simulink model "test"  (R2015a)
settings: Solver=ode45  StartTime=0.0  StopTime=380000  RelTol=1e-3
InitFcn:
  | %% DSPBuilder Start
  | alt_dspbuilder_update_model(bdroot)
  | %% DSPBuilder End
libraries: allblocks_alteradspbuilder2 x2155
(part 4 of 24)

== system test/octave2/compare_descriptor/get_distance5 ==
  hist_in1 : Inport
  hist_in2 : Inport  Port=2
  clken : Inport  Port=3
  BusSplitter : Subsystem
  BusSplitter1 : Subsystem
  Parallel Adder Subtractor : allblocks_alteradspbuilder2/Parallel Adder Subtractor  number_of_inputs=8  direction=+  use_pipeline=on  pipeline_display=3  phase_selection=1  use_ena=on  use_aclr=off  allowFloatingPointOverride=on  logOutputs=off  logFile=C:\Users\ASUS\Desktop\sift_fpga_final\Octave_2\tb_test\test_octave2_compare%5Fdescriptor_get%5Fdistance5_Parallel+Adder+Subtractor.fixedpointlog
  sub_GradOrian : Subsystem
  sub_GradOrian1 : Subsystem
  sub_GradOrian2 : Subsystem
  sub_GradOrian3 : Subsystem
  sub_GradOrian4 : Subsystem
  sub_GradOrian5 : Subsystem
  sub_GradOrian6 : Subsystem
  sub_GradOrian7 : Subsystem
  distance_out : Outport
  wires:
  hist_in2/1 -> [hist_in2]
  hist_in1/1 -> [hist_in1]
  [hist_in1] -> BusSplitter/1(data_in)
  [hist_in2] -> BusSplitter1/1(data_in)
  BusSplitter/1(bin1) -> [bin_11]
  BusSplitter/2(bin2) -> [bin_12]
  BusSplitter/3(bin3) -> [bin_13]
  BusSplitter/4(bin4) -> [bin_14]
  BusSplitter/5(bin5) -> [bin_15]
  BusSplitter/6(bin6) -> [bin_16]
  BusSplitter/7(bin7) -> [bin_17]
  BusSplitter/8(bin8) -> [bin_18]
  BusSplitter1/1(bin1) -> [bin_21]
  BusSplitter1/2(bin2) -> [bin_22]
  BusSplitter1/3(bin3) -> [bin_23]
  BusSplitter1/4(bin4) -> [bin_24]
  BusSplitter1/5(bin5) -> [bin_25]
  BusSplitter1/6(bin6) -> [bin_26]
  BusSplitter1/7(bin7) -> [bin_27]
  BusSplitter1/8(bin8) -> [bin_28]
  [bin_21] -> sub_GradOrian/2(bin2)
  [bin_11] -> sub_GradOrian/1(bin1)
  clken/1 -> [clken]
  [clken] -> sub_GradOrian/3(clken)
  sub_GradOrian/1(sub_bin) -> [sub_bin1]
  [bin_22] -> sub_GradOrian1/2(bin2)
  [bin_12] -> sub_GradOrian1/1(bin1)
  [clken] -> sub_GradOrian1/3(clken)
  sub_GradOrian1/1(sub_bin) -> [sub_bin2]
  [bin_23] -> sub_GradOrian2/2(bin2)
  [bin_13] -> sub_GradOrian2/1(bin1)
  [clken] -> sub_GradOrian2/3(clken)
  sub_GradOrian2/1(sub_bin) -> [sub_bin3]
  [bin_24] -> sub_GradOrian3/2(bin2)
  [bin_14] -> sub_GradOrian3/1(bin1)
  [clken] -> sub_GradOrian3/3(clken)
  sub_GradOrian3/1(sub_bin) -> [sub_bin4]
  [bin_25] -> sub_GradOrian4/2(bin2)
  [bin_15] -> sub_GradOrian4/1(bin1)
  [clken] -> sub_GradOrian4/3(clken)
  sub_GradOrian4/1(sub_bin) -> [sub_bin5]
  [bin_26] -> sub_GradOrian5/2(bin2)
  [bin_16] -> sub_GradOrian5/1(bin1)
  [clken] -> sub_GradOrian5/3(clken)
  sub_GradOrian5/1(sub_bin) -> [sub_bin6]
  [bin_27] -> sub_GradOrian6/2(bin2)
  [bin_17] -> sub_GradOrian6/1(bin1)
  [clken] -> sub_GradOrian6/3(clken)
  sub_GradOrian6/1(sub_bin) -> [sub_bin7]
  [bin_28] -> sub_GradOrian7/2(bin2)
  [bin_18] -> sub_GradOrian7/1(bin1)
  [clken] -> sub_GradOrian7/3(clken)
  sub_GradOrian7/1(sub_bin) -> [sub_bin8]
  [sub_bin1] -> Parallel Adder Subtractor/1
  [sub_bin2] -> Parallel Adder Subtractor/2
  [sub_bin3] -> Parallel Adder Subtractor/3
  [sub_bin4] -> Parallel Adder Subtractor/4
  [sub_bin5] -> Parallel Adder Subtractor/5
  [sub_bin6] -> Parallel Adder Subtractor/6
  [sub_bin7] -> Parallel Adder Subtractor/7
  [sub_bin8] -> Parallel Adder Subtractor/8
  [clken] -> Parallel Adder Subtractor/9
  Parallel Adder Subtractor/1 -> [distance_out]
  [distance_out] -> distance_out/1

== system test/octave2/compare_descriptor/get_distance6 ==
  hist_in1 : Inport
  hist_in2 : Inport  Port=2
  clken : Inport  Port=3
  BusSplitter : Subsystem
  BusSplitter1 : Subsystem
  Parallel Adder Subtractor : allblocks_alteradspbuilder2/Parallel Adder Subtractor  number_of_inputs=8  direction=+  use_pipeline=on  pipeline_display=3  phase_selection=1  use_ena=on  use_aclr=off  allowFloatingPointOverride=on  logOutputs=off  logFile=C:\Users\ASUS\Desktop\sift_fpga_final\Octave_2\tb_test\test_octave2_compare%5Fdescriptor_get%5Fdistance6_Parallel+Adder+Subtractor.fixedpointlog
  sub_GradOrian : Subsystem
  sub_GradOrian1 : Subsystem
  sub_GradOrian2 : Subsystem
  sub_GradOrian3 : Subsystem
  sub_GradOrian4 : Subsystem
  sub_GradOrian5 : Subsystem
  sub_GradOrian6 : Subsystem
  sub_GradOrian7 : Subsystem
  distance_out : Outport
  wires:
  hist_in2/1 -> [hist_in2]
  hist_in1/1 -> [hist_in1]
  [hist_in1] -> BusSplitter/1(data_in)
  [hist_in2] -> BusSplitter1/1(data_in)
  BusSplitter/1(bin1) -> [bin_11]
  BusSplitter/2(bin2) -> [bin_12]
  BusSplitter/3(bin3) -> [bin_13]
  BusSplitter/4(bin4) -> [bin_14]
  BusSplitter/5(bin5) -> [bin_15]
  BusSplitter/6(bin6) -> [bin_16]
  BusSplitter/7(bin7) -> [bin_17]
  BusSplitter/8(bin8) -> [bin_18]
  BusSplitter1/1(bin1) -> [bin_21]
  BusSplitter1/2(bin2) -> [bin_22]
  BusSplitter1/3(bin3) -> [bin_23]
  BusSplitter1/4(bin4) -> [bin_24]
  BusSplitter1/5(bin5) -> [bin_25]
  BusSplitter1/6(bin6) -> [bin_26]
  BusSplitter1/7(bin7) -> [bin_27]
  BusSplitter1/8(bin8) -> [bin_28]
  [bin_21] -> sub_GradOrian/2(bin2)
  [bin_11] -> sub_GradOrian/1(bin1)
  clken/1 -> [clken]
  [clken] -> sub_GradOrian/3(clken)
  sub_GradOrian/1(sub_bin) -> [sub_bin1]
  [bin_22] -> sub_GradOrian1/2(bin2)
  [bin_12] -> sub_GradOrian1/1(bin1)
  [clken] -> sub_GradOrian1/3(clken)
  sub_GradOrian1/1(sub_bin) -> [sub_bin2]
  [bin_23] -> sub_GradOrian2/2(bin2)
  [bin_13] -> sub_GradOrian2/1(bin1)
  [clken] -> sub_GradOrian2/3(clken)
  sub_GradOrian2/1(sub_bin) -> [sub_bin3]
  [bin_24] -> sub_GradOrian3/2(bin2)
  [bin_14] -> sub_GradOrian3/1(bin1)
  [clken] -> sub_GradOrian3/3(clken)
  sub_GradOrian3/1(sub_bin) -> [sub_bin4]
  [bin_25] -> sub_GradOrian4/2(bin2)
  [bin_15] -> sub_GradOrian4/1(bin1)
  [clken] -> sub_GradOrian4/3(clken)
  sub_GradOrian4/1(sub_bin) -> [sub_bin5]
  [bin_26] -> sub_GradOrian5/2(bin2)
  [bin_16] -> sub_GradOrian5/1(bin1)
  [clken] -> sub_GradOrian5/3(clken)
  sub_GradOrian5/1(sub_bin) -> [sub_bin6]
  [bin_27] -> sub_GradOrian6/2(bin2)
  [bin_17] -> sub_GradOrian6/1(bin1)
  [clken] -> sub_GradOrian6/3(clken)
  sub_GradOrian6/1(sub_bin) -> [sub_bin7]
  [bin_28] -> sub_GradOrian7/2(bin2)
  [bin_18] -> sub_GradOrian7/1(bin1)
  [clken] -> sub_GradOrian7/3(clken)
  sub_GradOrian7/1(sub_bin) -> [sub_bin8]
  [sub_bin1] -> Parallel Adder Subtractor/1
  [sub_bin2] -> Parallel Adder Subtractor/2
  [sub_bin3] -> Parallel Adder Subtractor/3
  [sub_bin4] -> Parallel Adder Subtractor/4
  [sub_bin5] -> Parallel Adder Subtractor/5
  [sub_bin6] -> Parallel Adder Subtractor/6
  [sub_bin7] -> Parallel Adder Subtractor/7
  [sub_bin8] -> Parallel Adder Subtractor/8
  [clken] -> Parallel Adder Subtractor/9
  Parallel Adder Subtractor/1 -> [distance_out]
  [distance_out] -> distance_out/1

== system test/octave2/compare_descriptor/get_distance7 ==
  hist_in1 : Inport
  hist_in2 : Inport  Port=2
  clken : Inport  Port=3
  BusSplitter : Subsystem
  BusSplitter1 : Subsystem
  Parallel Adder Subtractor : allblocks_alteradspbuilder2/Parallel Adder Subtractor  number_of_inputs=8  direction=+  use_pipeline=on  pipeline_display=3  phase_selection=1  use_ena=on  use_aclr=off  allowFloatingPointOverride=on  logOutputs=off  logFile=C:\Users\ASUS\Desktop\sift_fpga_final\Octave_2\tb_test\test_octave2_compare%5Fdescriptor_get%5Fdistance7_Parallel+Adder+Subtractor.fixedpointlog
  sub_GradOrian : Subsystem
  sub_GradOrian1 : Subsystem
  sub_GradOrian2 : Subsystem
  sub_GradOrian3 : Subsystem
  sub_GradOrian4 : Subsystem
  sub_GradOrian5 : Subsystem
  sub_GradOrian6 : Subsystem
  sub_GradOrian7 : Subsystem
  distance_out : Outport
  wires:
  hist_in2/1 -> [hist_in2]
  hist_in1/1 -> [hist_in1]
  [hist_in1] -> BusSplitter/1(data_in)
  [hist_in2] -> BusSplitter1/1(data_in)
  BusSplitter/1(bin1) -> [bin_11]
  BusSplitter/2(bin2) -> [bin_12]
  BusSplitter/3(bin3) -> [bin_13]
  BusSplitter/4(bin4) -> [bin_14]
  BusSplitter/5(bin5) -> [bin_15]
  BusSplitter/6(bin6) -> [bin_16]
  BusSplitter/7(bin7) -> [bin_17]
  BusSplitter/8(bin8) -> [bin_18]
  BusSplitter1/1(bin1) -> [bin_21]
  BusSplitter1/2(bin2) -> [bin_22]
  BusSplitter1/3(bin3) -> [bin_23]
  BusSplitter1/4(bin4) -> [bin_24]
  BusSplitter1/5(bin5) -> [bin_25]
  BusSplitter1/6(bin6) -> [bin_26]
  BusSplitter1/7(bin7) -> [bin_27]
  BusSplitter1/8(bin8) -> [bin_28]
  [bin_21] -> sub_GradOrian/2(bin2)
  [bin_11] -> sub_GradOrian/1(bin1)
  clken/1 -> [clken]
  [clken] -> sub_GradOrian/3(clken)
  sub_GradOrian/1(sub_bin) -> [sub_bin1]
  [bin_22] -> sub_GradOrian1/2(bin2)
  [bin_12] -> sub_GradOrian1/1(bin1)
  [clken] -> sub_GradOrian1/3(clken)
  sub_GradOrian1/1(sub_bin) -> [sub_bin2]
  [bin_23] -> sub_GradOrian2/2(bin2)
  [bin_13] -> sub_GradOrian2/1(bin1)
  [clken] -> sub_GradOrian2/3(clken)
  sub_GradOrian2/1(sub_bin) -> [sub_bin3]
  [bin_24] -> sub_GradOrian3/2(bin2)
  [bin_14] -> sub_GradOrian3/1(bin1)
  [clken] -> sub_GradOrian3/3(clken)
  sub_GradOrian3/1(sub_bin) -> [sub_bin4]
  [bin_25] -> sub_GradOrian4/2(bin2)
  [bin_15] -> sub_GradOrian4/1(bin1)
  [clken] -> sub_GradOrian4/3(clken)
  sub_GradOrian4/1(sub_bin) -> [sub_bin5]
  [bin_26] -> sub_GradOrian5/2(bin2)
  [bin_16] -> sub_GradOrian5/1(bin1)
  [clken] -> sub_GradOrian5/3(clken)
  sub_GradOrian5/1(sub_bin) -> [sub_bin6]
  [bin_27] -> sub_GradOrian6/2(bin2)
  [bin_17] -> sub_GradOrian6/1(bin1)
  [clken] -> sub_GradOrian6/3(clken)
  sub_GradOrian6/1(sub_bin) -> [sub_bin7]
  [bin_28] -> sub_GradOrian7/2(bin2)
  [bin_18] -> sub_GradOrian7/1(bin1)
  [clken] -> sub_GradOrian7/3(clken)
  sub_GradOrian7/1(sub_bin) -> [sub_bin8]
  [sub_bin1] -> Parallel Adder Subtractor/1
  [sub_bin2] -> Parallel Adder Subtractor/2
  [sub_bin3] -> Parallel Adder Subtractor/3
  [sub_bin4] -> Parallel Adder Subtractor/4
  [sub_bin5] -> Parallel Adder Subtractor/5
  [sub_bin6] -> Parallel Adder Subtractor/6
  [sub_bin7] -> Parallel Adder Subtractor/7
  [sub_bin8] -> Parallel Adder Subtractor/8
  [clken] -> Parallel Adder Subtractor/9
  Parallel Adder Subtractor/1 -> [distance_out]
  [distance_out] -> distance_out/1

== system test/octave2/compare_descriptor/get_distance8 ==
  hist_in1 : Inport
  hist_in2 : Inport  Port=2
  clken : Inport  Port=3
  BusSplitter : Subsystem
  BusSplitter1 : Subsystem
  Parallel Adder Subtractor : allblocks_alteradspbuilder2/Parallel Adder Subtractor  number_of_inputs=8  direction=+  use_pipeline=on  pipeline_display=3  phase_selection=1  use_ena=on  use_aclr=off  allowFloatingPointOverride=on  logOutputs=off  logFile=C:\Users\ASUS\Desktop\sift_fpga_final\Octave_2\tb_test\test_octave2_compare%5Fdescriptor_get%5Fdistance8_Parallel+Adder+Subtractor.fixedpointlog
  sub_GradOrian : Subsystem
  sub_GradOrian1 : Subsystem
  sub_GradOrian2 : Subsystem
  sub_GradOrian3 : Subsystem
  sub_GradOrian4 : Subsystem
  sub_GradOrian5 : Subsystem
  sub_GradOrian6 : Subsystem
  sub_GradOrian7 : Subsystem
  distance_out : Outport
  wires:
  hist_in2/1 -> [hist_in2]
  hist_in1/1 -> [hist_in1]
  [hist_in1] -> BusSplitter/1(data_in)
  [hist_in2] -> BusSplitter1/1(data_in)
  BusSplitter/1(bin1) -> [bin_11]
  BusSplitter/2(bin2) -> [bin_12]
  BusSplitter/3(bin3) -> [bin_13]
  BusSplitter/4(bin4) -> [bin_14]
  BusSplitter/5(bin5) -> [bin_15]
  BusSplitter/6(bin6) -> [bin_16]
  BusSplitter/7(bin7) -> [bin_17]
  BusSplitter/8(bin8) -> [bin_18]
  BusSplitter1/1(bin1) -> [bin_21]
  BusSplitter1/2(bin2) -> [bin_22]
  BusSplitter1/3(bin3) -> [bin_23]
  BusSplitter1/4(bin4) -> [bin_24]
  BusSplitter1/5(bin5) -> [bin_25]
  BusSplitter1/6(bin6) -> [bin_26]
  BusSplitter1/7(bin7) -> [bin_27]
  BusSplitter1/8(bin8) -> [bin_28]
  [bin_21] -> sub_GradOrian/2(bin2)
  [bin_11] -> sub_GradOrian/1(bin1)
  clken/1 -> [clken]
  [clken] -> sub_GradOrian/3(clken)
  sub_GradOrian/1(sub_bin) -> [sub_bin1]
  [bin_22] -> sub_GradOrian1/2(bin2)
  [bin_12] -> sub_GradOrian1/1(bin1)
  [clken] -> sub_GradOrian1/3(clken)
  sub_GradOrian1/1(sub_bin) -> [sub_bin2]
  [bin_23] -> sub_GradOrian2/2(bin2)
  [bin_13] -> sub_GradOrian2/1(bin1)
  [clken] -> sub_GradOrian2/3(clken)
  sub_GradOrian2/1(sub_bin) -> [sub_bin3]
  [bin_24] -> sub_GradOrian3/2(bin2)
  [bin_14] -> sub_GradOrian3/1(bin1)
  [clken] -> sub_GradOrian3/3(clken)
  sub_GradOrian3/1(sub_bin) -> [sub_bin4]
  [bin_25] -> sub_GradOrian4/2(bin2)
  [bin_15] -> sub_GradOrian4/1(bin1)
  [clken] -> sub_GradOrian4/3(clken)
  sub_GradOrian4/1(sub_bin) -> [sub_bin5]
  [bin_26] -> sub_GradOrian5/2(bin2)
  [bin_16] -> sub_GradOrian5/1(bin1)
  [clken] -> sub_GradOrian5/3(clken)
  sub_GradOrian5/1(sub_bin) -> [sub_bin6]
  [bin_27] -> sub_GradOrian6/2(bin2)
  [bin_17] -> sub_GradOrian6/1(bin1)
  [clken] -> sub_GradOrian6/3(clken)
  sub_GradOrian6/1(sub_bin) -> [sub_bin7]
  [bin_28] -> sub_GradOrian7/2(bin2)
  [bin_18] -> sub_GradOrian7/1(bin1)
  [clken] -> sub_GradOrian7/3(clken)
  sub_GradOrian7/1(sub_bin) -> [sub_bin8]
  [sub_bin1] -> Parallel Adder Subtractor/1
  [sub_bin2] -> Parallel Adder Subtractor/2
  [sub_bin3] -> Parallel Adder Subtractor/3
  [sub_bin4] -> Parallel Adder Subtractor/4
  [sub_bin5] -> Parallel Adder Subtractor/5
  [sub_bin6] -> Parallel Adder Subtractor/6
  [sub_bin7] -> Parallel Adder Subtractor/7
  [sub_bin8] -> Parallel Adder Subtractor/8
  [clken] -> Parallel Adder Subtractor/9
  Parallel Adder Subtractor/1 -> [distance_out]
  [distance_out] -> distance_out/1

== system test/octave2/descriptor/BusSplitter ==
  data_in : Inport
  AltBus : allblocks_alteradspbuilder2/AltBus  BusType=Unsigned Integer  bwl=112  bwr=0  saturate=off  floatingPointInput=on  floatingPointOutput=on  logOutputs=off  logFile=C:\Users\ASUS\Desktop\sift_fpga_final\Octave_2\tb_test\test_octave2_descriptor_BusSplitter_AltBus.fixedpointlog
  AltBus1 : allblocks_alteradspbuilder2/AltBus  BusType=Unsigned Integer  bwl=96  bwr=0  saturate=off  floatingPointInput=on  floatingPointOutput=on  logOutputs=off  logFile=C:\Users\ASUS\Desktop\sift_fpga_final\Octave_2\tb_test\test_octave2_descriptor_BusSplitter_AltBus1.fixedpointlog
  AltBus10 : allblocks_alteradspbuilder2/AltBus  BusType=Unsigned Integer  bwl=16  bwr=0  saturate=off  floatingPointInput=on  floatingPointOutput=on  logOutputs=off  logFile=C:\Users\ASUS\Desktop\sift_fpga_final\Octave_2\tb_test\test_octave2_descriptor_BusSplitter_AltBus10.fixedpointlog
  AltBus11 : allblocks_alteradspbuilder2/AltBus  BusType=Unsigned Integer  bwl=16  bwr=0  saturate=off  floatingPointInput=on  floatingPointOutput=on  logOutputs=off  logFile=C:\Users\ASUS\Desktop\sift_fpga_final\Octave_2\tb_test\test_octave2_descriptor_BusSplitter_AltBus11.fixedpointlog
  AltBus12 : allblocks_alteradspbuilder2/AltBus  BusType=Unsigned Integer  bwl=16  bwr=0  saturate=off  floatingPointInput=on  floatingPointOutput=on  logOutputs=off  logFile=C:\Users\ASUS\Desktop\sift_fpga_final\Octave_2\tb_test\test_octave2_descriptor_BusSplitter_AltBus12.fixedpointlog
  AltBus13 : allblocks_alteradspbuilder2/AltBus  BusType=Unsigned Integer  bwl=16  bwr=0  saturate=off  floatingPointInput=on  floatingPointOutput=on  logOutputs=off  logFile=C:\Users\ASUS\Desktop\sift_fpga_final\Octave_2\tb_test\test_octave2_descriptor_BusSplitter_AltBus13.fixedpointlog
  AltBus2 : allblocks_alteradspbuilder2/AltBus  BusType=Unsigned Integer  bwl=80  bwr=0  saturate=off  floatingPointInput=on  floatingPointOutput=on  logOutputs=off  logFile=C:\Users\ASUS\Desktop\sift_fpga_final\Octave_2\tb_test\test_octave2_descriptor_BusSplitter_AltBus2.fixedpointlog
  AltBus3 : allblocks_alteradspbuilder2/AltBus  BusType=Unsigned Integer  bwl=64  bwr=0  saturate=off  floatingPointInput=on  floatingPointOutput=on  logOutputs=off  logFile=C:\Users\ASUS\Desktop\sift_fpga_final\Octave_2\tb_test\test_octave2_descriptor_BusSplitter_AltBus3.fixedpointlog
  AltBus4 : allblocks_alteradspbuilder2/AltBus  BusType=Unsigned Integer  bwl=48  bwr=0  saturate=off  floatingPointInput=on  floatingPointOutput=on  logOutputs=off  logFile=C:\Users\ASUS\Desktop\sift_fpga_final\Octave_2\tb_test\test_octave2_descriptor_BusSplitter_AltBus4.fixedpointlog
  AltBus5 : allblocks_alteradspbuilder2/AltBus  BusType=Unsigned Integer  bwl=32  bwr=0  saturate=off  floatingPointInput=on  floatingPointOutput=on  logOutputs=off  logFile=C:\Users\ASUS\Desktop\sift_fpga_final\Octave_2\tb_test\test_octave2_descriptor_BusSplitter_AltBus5.fixedpointlog
  AltBus6 : allblocks_alteradspbuilder2/AltBus  BusType=Unsigned Integer  bwl=16  bwr=0  saturate=off  floatingPointInput=on  floatingPointOutput=on  logOutputs=off  logFile=C:\Users\ASUS\Desktop\sift_fpga_final\Octave_2\tb_test\test_octave2_descriptor_BusSplitter_AltBus6.fixedpointlog
  AltBus7 : allblocks_alteradspbuilder2/AltBus  BusType=Unsigned Integer  bwl=16  bwr=0  saturate=off  floatingPointInput=on  floatingPointOutput=on  logOutputs=off  logFile=C:\Users\ASUS\Desktop\sift_fpga_final\Octave_2\tb_test\test_octave2_descriptor_BusSplitter_AltBus7.fixedpointlog
  AltBus8 : allblocks_alteradspbuilder2/AltBus  BusType=Unsigned Integer  bwl=16  bwr=0  saturate=off  floatingPointInput=on  floatingPointOutput=on  logOutputs=off  logFile=C:\Users\ASUS\Desktop\sift_fpga_final\Octave_2\tb_test\test_octave2_descriptor_BusSplitter_AltBus8.fixedpointlog
  AltBus9 : allblocks_alteradspbuilder2/AltBus  BusType=Unsigned Integer  bwl=16  bwr=0  saturate=off  floatingPointInput=on  floatingPointOutput=on  logOutputs=off  logFile=C:\Users\ASUS\Desktop\sift_fpga_final\Octave_2\tb_test\test_octave2_descriptor_BusSplitter_AltBus9.fixedpointlog
  Logical Bus Operator : allblocks_alteradspbuilder2/Logical Bus Operator  BusType=Unsigned Integer  bwl=128  bwr=0  LogicalOp_text=Shift Right  mask_value_num=-5  shift_amount=112  force_sign_ext=off  pipeline_display=0
  Logical Bus Operator1 : allblocks_alteradspbuilder2/Logical Bus Operator  BusType=Unsigned Integer  bwl=112  bwr=0  LogicalOp_text=Shift Right  mask_value_num=-5  shift_amount=96  force_sign_ext=off  pipeline_display=0
  Logical Bus Operator2 : allblocks_alteradspbuilder2/Logical Bus Operator  BusType=Unsigned Integer  bwl=96  bwr=0  LogicalOp_text=Shift Right  mask_value_num=-5  shift_amount=80  force_sign_ext=off  pipeline_display=0
  Logical Bus Operator3 : allblocks_alteradspbuilder2/Logical Bus Operator  BusType=Unsigned Integer  bwl=80  bwr=0  LogicalOp_text=Shift Right  mask_value_num=-5  shift_amount=64  force_sign_ext=off  pipeline_display=0
  Logical Bus Operator4 : allblocks_alteradspbuilder2/Logical Bus Operator  BusType=Unsigned Integer  bwl=64  bwr=0  LogicalOp_text=Shift Right  mask_value_num=-5  shift_amount=48  force_sign_ext=off  pipeline_display=0
  Logical Bus Operator5 : allblocks_alteradspbuilder2/Logical Bus Operator  BusType=Unsigned Integer  bwl=48  bwr=0  LogicalOp_text=Shift Right  mask_value_num=-5  shift_amount=32  force_sign_ext=off  pipeline_display=0
  Logical Bus Operator6 : allblocks_alteradspbuilder2/Logical Bus Operator  BusType=Unsigned Integer  bwl=32  bwr=0  LogicalOp_text=Shift Right  mask_value_num=-5  shift_amount=16  force_sign_ext=off  pipeline_display=0
  bin1 : Outport
  bin2 : Outport  Port=2
  bin3 : Outport  Port=3
  bin4 : Outport  Port=4
  bin5 : Outport  Port=5
  bin6 : Outport  Port=6
  bin7 : Outport  Port=7
  bin8 : Outport  Port=8
  wires:
  Logical Bus Operator6/1 -> AltBus7/1
  AltBus1/1 -> Logical Bus Operator2/1
  AltBus9/1 -> bin5/1
  AltBus8/1 -> bin6/1
  AltBus7/1 -> bin7/1
  AltBus6/1 -> bin8/1
  AltBus/1 -> Logical Bus Operator1/1
  AltBus10/1 -> bin4/1
  AltBus12/1 -> bin3/1
  AltBus11/1 -> bin1/1
  AltBus3/1 -> Logical Bus Operator4/1
  AltBus2/1 -> Logical Bus Operator3/1
  AltBus4/1 -> Logical Bus Operator5/1
  data_in/1 -> AltBus6/1, AltBus5/1, AltBus4/1, AltBus3/1, AltBus2/1, AltBus1/1, AltBus/1, Logical Bus Operator/1
  AltBus5/1 -> Logical Bus Operator6/1
  Logical Bus Operator1/1 -> AltBus13/1
  Logical Bus Operator2/1 -> AltBus12/1
  Logical Bus Operator/1 -> AltBus11/1
  Logical Bus Operator5/1 -> AltBus8/1
  Logical Bus Operator4/1 -> AltBus9/1
  Logical Bus Operator3/1 -> AltBus10/1
  AltBus13/1 -> bin2/1

== system test/octave2/descriptor/descriptor ==
  data_in1 : Inport
  data_in2 : Inport  Port=2
  data_in3 : Inport  Port=3
  data_in4 : Inport  Port=4
  data_in5 : Inport  Port=5
  data_in6 : Inport  Port=6
  data_in7 : Inport  Port=7
  data_in8 : Inport  Port=8
  data_in9 : Inport  Port=9
  Bus Concatenation{68..69,76..77,84..85,92..93,100..101,104..105,112..113,120..121} (16 alike) : allblocks_alteradspbuilder2/Bus Concatenation  isSigned=off  awidth=256  bwidth=256  pipeline_display=0
  Bus Concatenation{70,78,86,94,102,106,114,122} (8 alike) : allblocks_alteradspbuilder2/Bus Concatenation  isSigned=off  awidth=512  bwidth=512  pipeline_display=0
  Bus Concatenation{71,79,87,95,103,107,115,123} (8 alike) : allblocks_alteradspbuilder2/Bus Concatenation  isSigned=off  awidth=128  bwidth=1024  pipeline_display=0
  Bus Concatenation{64..67,72..75,80..83,88..91,96..99,108..111,116..119,124..127} (32 alike) : allblocks_alteradspbuilder2/Bus Concatenation  isSigned=off  awidth=128  bwidth=128  pipeline_display=0
  descriptor1 : Outport
  descriptor2 : Outport  Port=2
  descriptor3 : Outport  Port=3
  descriptor4 : Outport  Port=4
  descriptor5 : Outport  Port=5
  descriptor6 : Outport  Port=6
  descriptor7 : Outport  Port=7
  descriptor8 : Outport  Port=8
  wires:
  data_in2/1 -> [hist_05]
  data_in4/1 -> [hist_50]
  data_in6/1 -> [hist_510]
  data_in5/1 -> [hist_55]
  data_in7/1 -> [hist_100]
  data_in8/1 -> [hist_105]
  data_in3/1 -> [hist_010]
  data_in1/1 -> [hist_00]
  data_in9/1 -> [hist_1010]
  [hist_1010] -> Bus Concatenation64/2
  [hist_105] -> Bus Concatenation64/1
  [hist_100] -> Bus Concatenation65/2
  [hist_50] -> Bus Concatenation65/1
  [hist_00] -> Bus Concatenation66/2
  [hist_05] -> Bus Concatenation66/1
  [hist_010] -> Bus Concatenation67/2
  [hist_510] -> Bus Concatenation67/1
  Bus Concatenation64/1 -> Bus Concatenation68/2
  Bus Concatenation65/1 -> Bus Concatenation68/1
  Bus Concatenation66/1 -> Bus Concatenation69/2
  Bus Concatenation67/1 -> Bus Concatenation69/1
  Bus Concatenation69/1 -> Bus Concatenation70/1
  Bus Concatenation68/1 -> Bus Concatenation70/2
  Bus Concatenation70/1 -> Bus Concatenation71/2
  [hist_55] -> Bus Concatenation71/1
  Bus Concatenation71/1 -> descriptor1/1
  Bus Concatenation72/1 -> Bus Concatenation76/2
  Bus Concatenation73/1 -> Bus Concatenation76/1
  Bus Concatenation74/1 -> Bus Concatenation77/2
  Bus Concatenation75/1 -> Bus Concatenation77/1
  Bus Concatenation77/1 -> Bus Concatenation78/1
  Bus Concatenation76/1 -> Bus Concatenation78/2
  Bus Concatenation78/1 -> Bus Concatenation79/2
  [hist_55] -> Bus Concatenation79/1
  Bus Concatenation79/1 -> descriptor2/1
  [hist_1010] -> Bus Concatenation72/1
  [hist_105] -> Bus Concatenation73/2
  [hist_100] -> Bus Concatenation73/1
  [hist_50] -> Bus Concatenation74/2
  [hist_00] -> Bus Concatenation74/1
  [hist_05] -> Bus Concatenation75/2
  [hist_010] -> Bus Concatenation75/1
  [hist_510] -> Bus Concatenation72/2
  Bus Concatenation80/1 -> Bus Concatenation84/2
  Bus Concatenation81/1 -> Bus Concatenation84/1
  Bus Concatenation82/1 -> Bus Concatenation85/2
  Bus Concatenation83/1 -> Bus Concatenation85/1
  Bus Concatenation85/1 -> Bus Concatenation86/1
  Bus Concatenation84/1 -> Bus Concatenation86/2
  Bus Concatenation86/1 -> Bus Concatenation87/2
  [hist_55] -> Bus Concatenation87/1
  Bus Concatenation87/1 -> descriptor3/1
  [hist_1010] -> Bus Concatenation81/2
  [hist_105] -> Bus Concatenation81/1
  [hist_100] -> Bus Concatenation82/2
  [hist_50] -> Bus Concatenation82/1
  [hist_00] -> Bus Concatenation83/2
  [hist_05] -> Bus Concatenation83/1
  [hist_010] -> Bus Concatenation80/2
  [hist_510] -> Bus Concatenation80/1
  Bus Concatenation88/1 -> Bus Concatenation92/2
  Bus Concatenation89/1 -> Bus Concatenation92/1
  Bus Concatenation90/1 -> Bus Concatenation93/2
  Bus Concatenation91/1 -> Bus Concatenation93/1
  Bus Concatenation93/1 -> Bus Concatenation94/1
  Bus Concatenation92/1 -> Bus Concatenation94/2
  Bus Concatenation94/1 -> Bus Concatenation95/2
  [hist_55] -> Bus Concatenation95/1
  Bus Concatenation95/1 -> descriptor4/1
  [hist_1010] -> Bus Concatenation89/1
  [hist_105] -> Bus Concatenation90/2
  [hist_100] -> Bus Concatenation90/1
  [hist_50] -> Bus Concatenation91/2
  [hist_00] -> Bus Concatenation91/1
  [hist_05] -> Bus Concatenation88/2
  [hist_010] -> Bus Concatenation88/1
  [hist_510] -> Bus Concatenation89/2
  Bus Concatenation96/1 -> Bus Concatenation100/2
  Bus Concatenation97/1 -> Bus Concatenation100/1
  Bus Concatenation98/1 -> Bus Concatenation101/2
  Bus Concatenation99/1 -> Bus Concatenation101/1
  Bus Concatenation101/1 -> Bus Concatenation102/1
  Bus Concatenation100/1 -> Bus Concatenation102/2
  Bus Concatenation102/1 -> Bus Concatenation103/2
  [hist_55] -> Bus Concatenation103/1
  Bus Concatenation103/1 -> descriptor5/1
  Bus Concatenation108/1 -> Bus Concatenation104/2
  Bus Concatenation109/1 -> Bus Concatenation104/1
  Bus Concatenation110/1 -> Bus Concatenation105/2
  Bus Concatenation111/1 -> Bus Concatenation105/1
  Bus Concatenation105/1 -> Bus Concatenation106/1
  Bus Concatenation104/1 -> Bus Concatenation106/2
  Bus Concatenation106/1 -> Bus Concatenation107/2
  [hist_55] -> Bus Concatenation107/1
  Bus Concatenation107/1 -> descriptor6/1
  [hist_1010] -> Bus Concatenation98/2
  [hist_105] -> Bus Concatenation98/1
  [hist_100] -> Bus Concatenation99/2
  [hist_50] -> Bus Concatenation99/1
  [hist_00] -> Bus Concatenation96/2
  [hist_05] -> Bus Concatenation96/1
  [hist_010] -> Bus Concatenation97/2
  [hist_510] -> Bus Concatenation97/1
  [hist_1010] -> Bus Concatenation110/1
  [hist_105] -> Bus Concatenation111/2
  [hist_100] -> Bus Concatenation111/1
  [hist_50] -> Bus Concatenation108/2
  [hist_00] -> Bus Concatenation108/1
  [hist_05] -> Bus Concatenation109/2
  [hist_010] -> Bus Concatenation109/1
  [hist_510] -> Bus Concatenation110/2
  Bus Concatenation116/1 -> Bus Concatenation112/2
  Bus Concatenation117/1 -> Bus Concatenation112/1
  Bus Concatenation118/1 -> Bus Concatenation113/2
  Bus Concatenation119/1 -> Bus Concatenation113/1
  Bus Concatenation113/1 -> Bus Concatenation114/1
  Bus Concatenation112/1 -> Bus Concatenation114/2
  Bus Concatenation114/1 -> Bus Concatenation115/2
  [hist_55] -> Bus Concatenation115/1
  Bus Concatenation115/1 -> descriptor7/1
  [hist_1010] -> Bus Concatenation119/2
  [hist_105] -> Bus Concatenation119/1
  [hist_100] -> Bus Concatenation116/2
  [hist_50] -> Bus Concatenation116/1
  [hist_00] -> Bus Concatenation117/2
  [hist_05] -> Bus Concatenation117/1
  [hist_010] -> Bus Concatenation118/2
  [hist_510] -> Bus Concatenation118/1
  Bus Concatenation124/1 -> Bus Concatenation120/2
  Bus Concatenation125/1 -> Bus Concatenation120/1
  Bus Concatenation126/1 -> Bus Concatenation121/2
  Bus Concatenation127/1 -> Bus Concatenation121/1
  Bus Concatenation121/1 -> Bus Concatenation122/1
  Bus Concatenation120/1 -> Bus Concatenation122/2
  Bus Concatenation122/1 -> Bus Concatenation123/2
  [hist_55] -> Bus Concatenation123/1
  Bus Concatenation123/1 -> descriptor8/1
  [hist_1010] -> Bus Concatenation127/1
  [hist_105] -> Bus Concatenation124/2
  [hist_100] -> Bus Concatenation124/1
  [hist_50] -> Bus Concatenation125/2
  [hist_00] -> Bus Concatenation125/1
  [hist_05] -> Bus Concatenation126/2
  [hist_010] -> Bus Concatenation126/1
  [hist_510] -> Bus Concatenation127/2

== system test/octave2/descriptor/findMax ==
  bin1 : Inport
  bin2 : Inport  Port=2
  bin3 : Inport  Port=3
  bin4 : Inport  Port=4
  bin5 : Inport  Port=5
  bin6 : Inport  Port=6
  bin7 : Inport  Port=7
  bin8 : Inport  Port=8
  Bitwise Logical Bus Operator{,1..6} (7 alike) : allblocks_alteradspbuilder2/Bitwise Logical Bus Operator  BusType=Unsigned Integer  bwl=3  bwr=0  LogicalOperator=OR  pipeline_display=0
  Comparator1 : allblocks_alteradspbuilder2/Comparator  direction=a < b  pipeline_display=0  allowFloatingPointOverride=on  logOutputs=off  logFile=C:\Users\ASUS\Desktop\sift_fpga_final\Octave_2\tb_test\test_octave2_descriptor_findMax_Comparator1.fixedpointlog
  Comparator10 : allblocks_alteradspbuilder2/Comparator  direction=a == b  pipeline_display=0  allowFloatingPointOverride=on  logOutputs=off  logFile=C:\Users\ASUS\Desktop\sift_fpga_final\Octave_2\tb_test\test_octave2_descriptor_findMax_Comparator10.fixedpointlog
  Comparator11 : allblocks_alteradspbuilder2/Comparator  direction=a == b  pipeline_display=0  allowFloatingPointOverride=on  logOutputs=off  logFile=C:\Users\ASUS\Desktop\sift_fpga_final\Octave_2\tb_test\test_octave2_descriptor_findMax_Comparator11.fixedpointlog
  Comparator12 : allblocks_alteradspbuilder2/Comparator  direction=a == b  pipeline_display=0  allowFloatingPointOverride=on  logOutputs=off  logFile=C:\Users\ASUS\Desktop\sift_fpga_final\Octave_2\tb_test\test_octave2_descriptor_findMax_Comparator12.fixedpointlog
  Comparator13 : allblocks_alteradspbuilder2/Comparator  direction=a == b  pipeline_display=0  allowFloatingPointOverride=on  logOutputs=off  logFile=C:\Users\ASUS\Desktop\sift_fpga_final\Octave_2\tb_test\test_octave2_descriptor_findMax_Comparator13.fixedpointlog
  Comparator14 : allblocks_alteradspbuilder2/Comparator  direction=a == b  pipeline_display=0  allowFloatingPointOverride=on  logOutputs=off  logFile=C:\Users\ASUS\Desktop\sift_fpga_final\Octave_2\tb_test\test_octave2_descriptor_findMax_Comparator14.fixedpointlog
  Comparator19 : allblocks_alteradspbuilder2/Comparator  direction=a < b  pipeline_display=0  allowFloatingPointOverride=on  logOutputs=off  logFile=C:\Users\ASUS\Desktop\sift_fpga_final\Octave_2\tb_test\test_octave2_descriptor_findMax_Comparator19.fixedpointlog
  Comparator2 : allblocks_alteradspbuilder2/Comparator  direction=a < b  pipeline_display=0  allowFloatingPointOverride=on  logOutputs=off  logFile=C:\Users\ASUS\Desktop\sift_fpga_final\Octave_2\tb_test\test_octave2_descriptor_findMax_Comparator2.fixedpointlog
  Comparator3 : allblocks_alteradspbuilder2/Comparator  direction=a < b  pipeline_display=0  allowFloatingPointOverride=on  logOutputs=off  logFile=C:\Users\ASUS\Desktop\sift_fpga_final\Octave_2\tb_test\test_octave2_descriptor_findMax_Comparator3.fixedpointlog
  Comparator4 : allblocks_alteradspbuilder2/Comparator  direction=a < b  pipeline_display=0  allowFloatingPointOverride=on  logOutputs=off  logFile=C:\Users\ASUS\Desktop\sift_fpga_final\Octave_2\tb_test\test_octave2_descriptor_findMax_Comparator4.fixedpointlog
  Comparator5 : allblocks_alteradspbuilder2/Comparator  direction=a < b  pipeline_display=0  allowFloatingPointOverride=on  logOutputs=off  logFile=C:\Users\ASUS\Desktop\sift_fpga_final\Octave_2\tb_test\test_octave2_descriptor_findMax_Comparator5.fixedpointlog
  Comparator6 : allblocks_alteradspbuilder2/Comparator  direction=a < b  pipeline_display=0  allowFloatingPointOverride=on  logOutputs=off  logFile=C:\Users\ASUS\Desktop\sift_fpga_final\Octave_2\tb_test\test_octave2_descriptor_findMax_Comparator6.fixedpointlog
  Comparator7 : allblocks_alteradspbuilder2/Comparator  direction=a == b  pipeline_display=0  allowFloatingPointOverride=on  logOutputs=off  logFile=C:\Users\ASUS\Desktop\sift_fpga_final\Octave_2\tb_test\test_octave2_descriptor_findMax_Comparator7.fixedpointlog
  Comparator8 : allblocks_alteradspbuilder2/Comparator  direction=a == b  pipeline_display=0  allowFloatingPointOverride=on  logOutputs=off  logFile=C:\Users\ASUS\Desktop\sift_fpga_final\Octave_2\tb_test\test_octave2_descriptor_findMax_Comparator8.fixedpointlog
  Comparator9 : allblocks_alteradspbuilder2/Comparator  direction=a == b  pipeline_display=0  allowFloatingPointOverride=on  logOutputs=off  logFile=C:\Users\ASUS\Desktop\sift_fpga_final\Octave_2\tb_test\test_octave2_descriptor_findMax_Comparator9.fixedpointlog
  Constant10 : allblocks_alteradspbuilder2/Constant  mask_cst=0  BusType=Unsigned Integer  bwl=3  bwr=0  roundMode=Truncate  satMode=Wrap  SpecifyClock=off  allowFloatingPointOverride=on  logOutputs=off  logFile=C:\Users\ASUS\Desktop\sift_fpga_final\Octave_2\tb_test\test_octave2_descriptor_findMax_Constant10.fixedpointlog
  Constant11 : allblocks_alteradspbuilder2/Constant  mask_cst=1  BusType=Unsigned Integer  bwl=3  bwr=0  roundMode=Truncate  satMode=Wrap  SpecifyClock=off  allowFloatingPointOverride=on  logOutputs=off  logFile=C:\Users\ASUS\Desktop\sift_fpga_final\Octave_2\tb_test\test_octave2_descriptor_findMax_Constant11.fixedpointlog
  Constant12 : allblocks_alteradspbuilder2/Constant  mask_cst=0  BusType=Unsigned Integer  bwl=3  bwr=0  roundMode=Truncate  satMode=Wrap  SpecifyClock=off  allowFloatingPointOverride=on  logOutputs=off  logFile=C:\Users\ASUS\Desktop\sift_fpga_final\Octave_2\tb_test\test_octave2_descriptor_findMax_Constant12.fixedpointlog
  Constant13 : allblocks_alteradspbuilder2/Constant  mask_cst=3  BusType=Unsigned Integer  bwl=3  bwr=0  roundMode=Truncate  satMode=Wrap  SpecifyClock=off  allowFloatingPointOverride=on  logOutputs=off  logFile=C:\Users\ASUS\Desktop\sift_fpga_final\Octave_2\tb_test\test_octave2_descriptor_findMax_Constant13.fixedpointlog
  Constant14 : allblocks_alteradspbuilder2/Constant  mask_cst=0  BusType=Unsigned Integer  bwl=3  bwr=0  roundMode=Truncate  satMode=Wrap  SpecifyClock=off  allowFloatingPointOverride=on  logOutputs=off  logFile=C:\Users\ASUS\Desktop\sift_fpga_final\Octave_2\tb_test\test_octave2_descriptor_findMax_Constant14.fixedpointlog
  Constant15 : allblocks_alteradspbuilder2/Constant  mask_cst=2  BusType=Unsigned Integer  bwl=3  bwr=0  roundMode=Truncate  satMode=Wrap  SpecifyClock=off  allowFloatingPointOverride=on  logOutputs=off  logFile=C:\Users\ASUS\Desktop\sift_fpga_final\Octave_2\tb_test\test_octave2_descriptor_findMax_Constant15.fixedpointlog
  Constant16 : allblocks_alteradspbuilder2/Constant  mask_cst=0  BusType=Unsigned Integer  bwl=3  bwr=0  roundMode=Truncate  satMode=Wrap  SpecifyClock=off  allowFloatingPointOverride=on  logOutputs=off  logFile=C:\Users\ASUS\Desktop\sift_fpga_final\Octave_2\tb_test\test_octave2_descriptor_findMax_Constant16.fixedpointlog
  Constant17 : allblocks_alteradspbuilder2/Constant  mask_cst=5  BusType=Unsigned Integer  bwl=3  bwr=0  roundMode=Truncate  satMode=Wrap  SpecifyClock=off  allowFloatingPointOverride=on  logOutputs=off  logFile=C:\Users\ASUS\Desktop\sift_fpga_final\Octave_2\tb_test\test_octave2_descriptor_findMax_Constant17.fixedpointlog
  Constant18 : allblocks_alteradspbuilder2/Constant  mask_cst=0  BusType=Unsigned Integer  bwl=3  bwr=0  roundMode=Truncate  satMode=Wrap  SpecifyClock=off  allowFloatingPointOverride=on  logOutputs=off  logFile=C:\Users\ASUS\Desktop\sift_fpga_final\Octave_2\tb_test\test_octave2_descriptor_findMax_Constant18.fixedpointlog
  Constant19 : allblocks_alteradspbuilder2/Constant  mask_cst=7  BusType=Unsigned Integer  bwl=3  bwr=0  roundMode=Truncate  satMode=Wrap  SpecifyClock=off  allowFloatingPointOverride=on  logOutputs=off  logFile=C:\Users\ASUS\Desktop\sift_fpga_final\Octave_2\tb_test\test_octave2_descriptor_findMax_Constant19.fixedpointlog
  Constant20 : allblocks_alteradspbuilder2/Constant  mask_cst=0  BusType=Unsigned Integer  bwl=3  bwr=0  roundMode=Truncate  satMode=Wrap  SpecifyClock=off  allowFloatingPointOverride=on  logOutputs=off  logFile=C:\Users\ASUS\Desktop\sift_fpga_final\Octave_2\tb_test\test_octave2_descriptor_findMax_Constant20.fixedpointlog
  Constant21 : allblocks_alteradspbuilder2/Constant  mask_cst=6  BusType=Unsigned Integer  bwl=3  bwr=0  roundMode=Truncate  satMode=Wrap  SpecifyClock=off  allowFloatingPointOverride=on  logOutputs=off  logFile=C:\Users\ASUS\Desktop\sift_fpga_final\Octave_2\tb_test\test_octave2_descriptor_findMax_Constant21.fixedpointlog
  Constant22 : allblocks_alteradspbuilder2/Constant  mask_cst=0  BusType=Unsigned Integer  bwl=3  bwr=0  roundMode=Truncate  satMode=Wrap  SpecifyClock=off  allowFloatingPointOverride=on  logOutputs=off  logFile=C:\Users\ASUS\Desktop\sift_fpga_final\Octave_2\tb_test\test_octave2_descriptor_findMax_Constant22.fixedpointlog
  Constant23 : allblocks_alteradspbuilder2/Constant  mask_cst=4  BusType=Unsigned Integer  bwl=3  bwr=0  roundMode=Truncate  satMode=Wrap  SpecifyClock=off  allowFloatingPointOverride=on  logOutputs=off  logFile=C:\Users\ASUS\Desktop\sift_fpga_final\Octave_2\tb_test\test_octave2_descriptor_findMax_Constant23.fixedpointlog
  Constant8 : allblocks_alteradspbuilder2/Constant  mask_cst=0  BusType=Unsigned Integer  bwl=3  bwr=0  roundMode=Truncate  satMode=Wrap  SpecifyClock=off  allowFloatingPointOverride=on  logOutputs=off  logFile=C:\Users\ASUS\Desktop\sift_fpga_final\Octave_2\tb_test\test_octave2_descriptor_findMax_Constant8.fixedpointlog
  Constant9 : allblocks_alteradspbuilder2/Constant  mask_cst=0  BusType=Unsigned Integer  bwl=3  bwr=0  roundMode=Truncate  satMode=Wrap  SpecifyClock=off  allowFloatingPointOverride=on  logOutputs=off  logFile=C:\Users\ASUS\Desktop\sift_fpga_final\Octave_2\tb_test\test_octave2_descriptor_findMax_Constant9.fixedpointlog
  Multiplexer1 : allblocks_alteradspbuilder2/Multiplexer  numInputs=2  pipeline=0  oneHot=off  pipeline_display=0  use_ena=off  use_aclr=off  allowFloatingPointOverride=on  logOutputs=off  logFile=C:\Users\ASUS\Desktop\sift_fpga_final\Octave_2\tb_test\test_octave2_descriptor_findMax_Multiplexer1.fixedpointlog
  Multiplexer10 : allblocks_alteradspbuilder2/Multiplexer  numInputs=2  pipeline=0  oneHot=off  pipeline_display=0  use_ena=off  use_aclr=off  allowFloatingPointOverride=on  logOutputs=off  logFile=C:\Users\ASUS\Desktop\sift_fpga_final\Octave_2\tb_test\test_octave2_descriptor_findMax_Multiplexer10.fixedpointlog
  Multiplexer11 : allblocks_alteradspbuilder2/Multiplexer  numInputs=2  pipeline=0  oneHot=off  pipeline_display=0  use_ena=off  use_aclr=off  allowFloatingPointOverride=on  logOutputs=off  logFile=C:\Users\ASUS\Desktop\sift_fpga_final\Octave_2\tb_test\test_octave2_descriptor_findMax_Multiplexer11.fixedpointlog
  Multiplexer12 : allblocks_alteradspbuilder2/Multiplexer  numInputs=2  pipeline=0  oneHot=off  pipeline_display=0  use_ena=off  use_aclr=off  allowFloatingPointOverride=on  logOutputs=off  logFile=C:\Users\ASUS\Desktop\sift_fpga_final\Octave_2\tb_test\test_octave2_descriptor_findMax_Multiplexer12.fixedpointlog
  Multiplexer13 : allblocks_alteradspbuilder2/Multiplexer  numInputs=2  pipeline=0  oneHot=off  pipeline_display=0  use_ena=off  use_aclr=off  allowFloatingPointOverride=on  logOutputs=off  logFile=C:\Users\ASUS\Desktop\sift_fpga_final\Octave_2\tb_test\test_octave2_descriptor_findMax_Multiplexer13.fixedpointlog
  Multiplexer14 : allblocks_alteradspbuilder2/Multiplexer  numInputs=2  pipeline=0  oneHot=off  pipeline_display=0  use_ena=off  use_aclr=off  allowFloatingPointOverride=on  logOutputs=off  logFile=C:\Users\ASUS\Desktop\sift_fpga_final\Octave_2\tb_test\test_octave2_descriptor_findMax_Multiplexer14.fixedpointlog
  Multiplexer2 : allblocks_alteradspbuilder2/Multiplexer  numInputs=2  pipeline=0  oneHot=off  pipeline_display=0  use_ena=off  use_aclr=off  allowFloatingPointOverride=on  logOutputs=off  logFile=C:\Users\ASUS\Desktop\sift_fpga_final\Octave_2\tb_test\test_octave2_descriptor_findMax_Multiplexer2.fixedpointlog
  Multiplexer20 : allblocks_alteradspbuilder2/Multiplexer  numInputs=2  pipeline=0  oneHot=off  pipeline_display=0  use_ena=off  use_aclr=off  allowFloatingPointOverride=on  logOutputs=off  logFile=C:\Users\ASUS\Desktop\sift_fpga_final\Octave_2\tb_test\test_octave2_descriptor_findMax_Multiplexer20.fixedpointlog
  Multiplexer3 : allblocks_alteradspbuilder2/Multiplexer  numInputs=2  pipeline=0  oneHot=off  pipeline_display=0  use_ena=off  use_aclr=off  allowFloatingPointOverride=on  logOutputs=off  logFile=C:\Users\ASUS\Desktop\sift_fpga_final\Octave_2\tb_test\test_octave2_descriptor_findMax_Multiplexer3.fixedpointlog
  Multiplexer4 : allblocks_alteradspbuilder2/Multiplexer  numInputs=2  pipeline=0  oneHot=off  pipeline_display=0  use_ena=off  use_aclr=off  allowFloatingPointOverride=on  logOutputs=off  logFile=C:\Users\ASUS\Desktop\sift_fpga_final\Octave_2\tb_test\test_octave2_descriptor_findMax_Multiplexer4.fixedpointlog
  Multiplexer5 : allblocks_alteradspbuilder2/Multiplexer  numInputs=2  pipeline=0  oneHot=off  pipeline_display=0  use_ena=off  use_aclr=off  allowFloatingPointOverride=on  logOutputs=off  logFile=C:\Users\ASUS\Desktop\sift_fpga_final\Octave_2\tb_test\test_octave2_descriptor_findMax_Multiplexer5.fixedpointlog
  Multiplexer6 : allblocks_alteradspbuilder2/Multiplexer  numInputs=2  pipeline=0  oneHot=off  pipeline_display=0  use_ena=off  use_aclr=off  allowFloatingPointOverride=on  logOutputs=off  logFile=C:\Users\ASUS\Desktop\sift_fpga_final\Octave_2\tb_test\test_octave2_descriptor_findMax_Multiplexer6.fixedpointlog
  Multiplexer7 : allblocks_alteradspbuilder2/Multiplexer  numInputs=2  pipeline=0  oneHot=off  pipeline_display=0  use_ena=off  use_aclr=off  allowFloatingPointOverride=on  logOutputs=off  logFile=C:\Users\ASUS\Desktop\sift_fpga_final\Octave_2\tb_test\test_octave2_descriptor_findMax_Multiplexer7.fixedpointlog
  Multiplexer8 : allblocks_alteradspbuilder2/Multiplexer  numInputs=2  pipeline=0  oneHot=off  pipeline_display=0  use_ena=off  use_aclr=off  allowFloatingPointOverride=on  logOutputs=off  logFile=C:\Users\ASUS\Desktop\sift_fpga_final\Octave_2\tb_test\test_octave2_descriptor_findMax_Multiplexer8.fixedpointlog
  Multiplexer9 : allblocks_alteradspbuilder2/Multiplexer  numInputs=2  pipeline=0  oneHot=off  pipeline_display=0  use_ena=off  use_aclr=off  allowFloatingPointOverride=on  logOutputs=off  logFile=C:\Users\ASUS\Desktop\sift_fpga_final\Octave_2\tb_test\test_octave2_descriptor_findMax_Multiplexer9.fixedpointlog
  bin_max : Outport
  wires:
  [bin1] -> Comparator19/1
  [bin2] -> Comparator19/2
  Comparator19/1 -> Multiplexer20/1
  [bin1] -> Multiplexer20/2
  [bin2] -> Multiplexer20/3
  Multiplexer20/1 -> Comparator4/1, Multiplexer4/2
  [bin3] -> Comparator1/1
  [bin4] -> Comparator1/2
  Comparator1/1 -> Multiplexer1/1
  [bin3] -> Multiplexer1/2
  [bin4] -> Multiplexer1/3
  Multiplexer1/1 -> Multiplexer4/3, Comparator4/2
  [bin5] -> Comparator3/1
  [bin6] -> Comparator3/2
  Comparator3/1 -> Multiplexer3/1
  [bin5] -> Multiplexer3/2
  [bin6] -> Multiplexer3/3
  Multiplexer3/1 -> Comparator5/1, Multiplexer5/2
  [bin7] -> Comparator2/1
  [bin8] -> Comparator2/2
  Comparator2/1 -> Multiplexer2/1
  [bin7] -> Multiplexer2/2
  [bin8] -> Multiplexer2/3
  Multiplexer2/1 -> Multiplexer5/3, Comparator5/2
  Comparator4/1 -> Multiplexer4/1
  Comparator5/1 -> Multiplexer5/1
  Multiplexer4/1 -> Multiplexer6/2, Comparator6/1
  Multiplexer5/1 -> Comparator6/2, Multiplexer6/3
  Comparator6/1 -> Multiplexer6/1
  bin1/1 -> [bin1]
  bin2/1 -> [bin2]
  bin3/1 -> [bin3]
  bin4/1 -> [bin4]
  bin5/1 -> [bin5]
  bin6/1 -> [bin6]
  bin7/1 -> [bin7]
  bin8/1 -> [bin8]
  Bitwise Logical Bus Operator6/1 -> bin_max/1
  Multiplexer6/1 -> [binMax]
  [binMax] -> Comparator7/1
  [bin1] -> Comparator7/2
  Comparator7/1 -> Multiplexer7/1
  [binMax] -> Comparator8/1
  [bin2] -> Comparator8/2
  [binMax] -> Comparator9/1
  [bin3] -> Comparator9/2
  [binMax] -> Comparator10/1
  [bin4] -> Comparator10/2
  [binMax] -> Comparator12/1
  [bin5] -> Comparator12/2
  [binMax] -> Comparator13/1
  [bin6] -> Comparator13/2
  [binMax] -> Comparator14/1
  [bin7] -> Comparator14/2
  [binMax] -> Comparator11/1
  [bin8] -> Comparator11/2
  Constant8/1 -> Multiplexer7/2
  Constant9/1 -> Multiplexer7/3
  Comparator8/1 -> Multiplexer8/1
  Constant10/1 -> Multiplexer8/2
  Constant11/1 -> Multiplexer8/3
  Comparator9/1 -> Multiplexer9/1
  Constant14/1 -> Multiplexer9/2
  Constant15/1 -> Multiplexer9/3
  Comparator10/1 -> Multiplexer10/1
  Constant12/1 -> Multiplexer10/2
  Constant13/1 -> Multiplexer10/3
  Comparator12/1 -> Multiplexer12/1
  Constant22/1 -> Multiplexer12/2
  Constant23/1 -> Multiplexer12/3
  Comparator13/1 -> Multiplexer13/1
  Constant16/1 -> Multiplexer13/2
  Constant17/1 -> Multiplexer13/3
  Comparator14/1 -> Multiplexer14/1
  Constant20/1 -> Multiplexer14/2
  Constant21/1 -> Multiplexer14/3
  Comparator11/1 -> Multiplexer11/1
  Constant18/1 -> Multiplexer11/2
  Constant19/1 -> Multiplexer11/3
  Multiplexer7/1 -> Bitwise Logical Bus Operator/1
  Multiplexer8/1 -> Bitwise Logical Bus Operator/2
  Multiplexer9/1 -> Bitwise Logical Bus Operator1/1
  Multiplexer10/1 -> Bitwise Logical Bus Operator1/2
  Multiplexer12/1 -> Bitwise Logical Bus Operator2/1
  Multiplexer13/1 -> Bitwise Logical Bus Operator2/2
  Multiplexer14/1 -> Bitwise Logical Bus Operator3/1
  Multiplexer11/1 -> Bitwise Logical Bus Operator3/2
  Bitwise Logical Bus Operator/1 -> Bitwise Logical Bus Operator4/1
  Bitwise Logical Bus Operator1/1 -> Bitwise Logical Bus Operator4/2
  Bitwise Logical Bus Operator2/1 -> Bitwise Logical Bus Operator5/1
  Bitwise Logical Bus Operator3/1 -> Bitwise Logical Bus Operator5/2
  Bitwise Logical Bus Operator4/1 -> Bitwise Logical Bus Operator6/1
  Bitwise Logical Bus Operator5/1 -> Bitwise Logical Bus Operator6/2
